simulink model "CtrPlatform_AdaptiveControl"  (Simulink 7.9)
settings: Solver=ode3  StartTime=0.0  StopTime=8  FixedStep=Ts  RelTol=1e-3
InitFcn:
  | eval('CtrPlatformCfg')
StopFcn:
  | eval('CtrPlotTrj')
values from neighbouring files (symbols this model uses):
  A = [a1 a2 a3 a4 a5 a6]/180*pi    [Config.m]    (also in CtrPlatformCfg.m)
  a2 = 0    [Config.m]    (also in CtrPlatformCfg.m)
  a3 = 0    [Config.m]    (also in CtrPlatformCfg.m)
  a4 = 0    [Config.m]    (also in CtrPlatformCfg.m)
  a5 = 90    [Config.m]    (also in CtrPlatformCfg.m)
  a6 = 0    [Config.m]    (also in CtrPlatformCfg.m)
  Cen = Cen(:)'    [Config.m]    (also in CtrPlatformCfg.m; DynEulerTest.m = Cen'; EfDynCAD.m = [cen1,cen2,cen3,cen4,cen5,cen6]')
  CurPulseFreq = 0.25*2*pi    (= 1.57079632679)    [Config.m]    (also in CtrPlatformCfg.m)
  Deg2Rad = pi/180    (= 0.0174532925199)    [Config.m]    (also in CtrPlatformCfg.m)
  DisturbSelect = 2    [Config.m]    (also in CtrPlatformCfg.m)
  DynTrjMode = 3    [Config.m]    (also in CtrPlatformCfg.m = 1)
  FbDisturbSelect = 2    [Config.m]    (also in CtrPlatformCfg.m)
  freq = tvel/radius    (= 1)    [Config.m]    (also in CtrPlatformCfg.m)
  FrictionSelect = 2    [CtrPlatformCfg.m]
  Gravity = 9.8    [Config.m]    (also in CtrPlatformCfg.m)
  Ie1 = in1(:)'    [Config.m]    (also in CtrPlatformCfg.m; DynEulerTest.m = in1(:); EfDynCAD.m = in1(:))
  Ie2 = in2(:)'    [Config.m]    (also in CtrPlatformCfg.m; DynEulerTest.m = in2(:); EfDynCAD.m = in2(:))
  Ie3 = in3(:)'    [Config.m]    (also in CtrPlatformCfg.m; DynEulerTest.m = in3(:); EfDynCAD.m = in3(:))
  Ie4 = in4(:)'    [Config.m]    (also in CtrPlatformCfg.m; DynEulerTest.m = in4(:); EfDynCAD.m = in4(:))
  Ie5 = in5(:)'    [Config.m]    (also in CtrPlatformCfg.m; DynEulerTest.m = in5(:); EfDynCAD.m = in5(:))
  Ie6 = in6(:)'    [Config.m]    (also in CtrPlatformCfg.m; DynEulerTest.m = in6(:); EfDynCAD.m = in6(:))
  in1 = [5.2954 -0.2565 -0.6366;-0.2565 4.7000 0.2830;-0.6366 0.2829 5.8635]    [Config.m]    (also in CtrPlatformCfg.m; DynEulerTest.m; EfDynCAD.m = [0.54  -0.01 0.23)
  in2 = [5.8840 0.0072 0.0135;0.0072 6.0178 -0.1907;0.0135 -0.1907 0.3374]    [Config.m]    (also in CtrPlatformCfg.m; DynEulerTest.m; EfDynCAD.m = (R_x*R_z)*in2*(R_x*R_z)')
  in3 = [1.8201 -0.2274 -0.3112;-0.2274 2.2537 -0.1441;-0.3112 -0.1441 1.9485]    [Config.m]    (also in CtrPlatformCfg.m; DynEulerTest.m; EfDynCAD.m = (R_x*R_z)*in3*(R_x*R_z)')
  in4 = [0.0607 -0.0922 0;-0.0922 1.4493 0;0 0 1.4620]    [Config.m]    (also in CtrPlatformCfg.m; DynEulerTest.m = [0.0607 -0.0922 0;-0.0922 1.4493 0;0 0,1.4620]; EfDynCAD.m = (R_y*Rz)*in4*(R_y*Rz)')
  in5 = [0.0191 0.0032 0;0.0032 0.0228 0;0 0 0.0291]    [Config.m]    (also in CtrPlatformCfg.m; DynEulerTest.m; EfDynCAD.m = (R_x*R_y)*in5*(R_x*R_y)')
  in6 = [0.0012 0 0;0 0.0007 0;0 0 0.0007]    [Config.m]    (also in CtrPlatformCfg.m; DynEulerTest.m; EfDynCAD.m = (R_y*Rz)*in6*(R_y*Rz)')
  init_Endx = gd_init(1,4)    [Config.m]    (also in CtrPlatformCfg.m)
  init_Endy = gd_init(2,4)    [Config.m]    (also in CtrPlatformCfg.m)
  init_Endz = gd_init(3,4)    [Config.m]    (also in CtrPlatformCfg.m)
  init_Rot = gd_init(1:3,1:3)    [Config.m]    (also in CtrPlatformCfg.m)
  InitialPos1 = A(1)*Rad2Line(1)    [CtrPlatformCfg.m]
  InitialPos2 = A(2)*Rad2Line(2)    [CtrPlatformCfg.m]
  InitialPos3 = A(3)*Rad2Line(3)    [CtrPlatformCfg.m]
  InitialPos4 = A(4)*Rad2Line(4)    [CtrPlatformCfg.m]
  InitialPos5 = A(5)*Rad2Line(5)    [CtrPlatformCfg.m]
  InitialPos6 = A(6)*Rad2Line(6)    [CtrPlatformCfg.m]
  JntOffset1 = A(1)    [Config.m]    (also in CtrPlatformCfg.m)
  JntOffset2 = A(2)    [Config.m]    (also in CtrPlatformCfg.m)
  JntOffset3 = A(3)    [Config.m]    (also in CtrPlatformCfg.m)
  JntOffset4 = A(4)    [Config.m]    (also in CtrPlatformCfg.m)
  JntOffset5 = A(5)    [Config.m]    (also in CtrPlatformCfg.m)
  JntOffset6 = A(6)    [Config.m]    (also in CtrPlatformCfg.m)
  L = [l1 l2 l3 l4 l5 l6 l7 l8 l9]    [Config.m]    (also in CtrPlatformCfg.m)
  LinePTs2RadpS = 2*pi/(EncRes*Ts)./Gear    [Config.m]    (also in CtrPlatformCfg.m)
  LinePTs2Rpm = 60/(EncRes*Ts)    (= 7.32421875)    [Config.m]    (also in CtrPlatformCfg.m)
  Ma = [ma1 ma2 ma3 ma4 ma5 ma6]    [Config.m]    (also in CtrPlatformCfg.m; DynEulerTest.m = [ma1; ma2; ma3; ma4; ma5; ma6]; EfDynCAD.m = [ma1 ma2 ma3 ma4 ma5 ma6]')
  ma1 = 170.31    [Config.m]    (also in CtrPlatformCfg.m; DynEulerTest.m; EfDynCAD.m = 77.75)
  ma2 = 63.74    [Config.m]    (also in CtrPlatformCfg.m; DynEulerTest.m; EfDynCAD.m = 32.31)
  ma3 = 98.98    [Config.m]    (also in CtrPlatformCfg.m; DynEulerTest.m; EfDynCAD.m = 18.61)
  ma4 = 24.46    [Config.m]    (also in CtrPlatformCfg.m; DynEulerTest.m; EfDynCAD.m = 15.65)
  ma5 = 5.24    [Config.m]    (also in CtrPlatformCfg.m; DynEulerTest.m; EfDynCAD.m = 3.32)
  ma6 = 0.6    [Config.m]    (also in CtrPlatformCfg.m; DynEulerTest.m; EfDynCAD.m)
  Pi0 = PiTest    [CtrPlatformCfg.m]
  PosPulseEnable = 1    [Config.m]    (also in CtrPlatformCfg.m)
  PosSourceSelect_Ad = 2    [CtrPlatformCfg.m]
  PosVelPulseGain = 500    [Config.m]    (also in CtrPlatformCfg.m)
  Rad2Line = Gear*EncRes/(2*pi)    [Config.m]    (also in CtrPlatformCfg.m)
  Rpm2LinePTs = EncRes*Ts/60    (= 0.136533333333)    [Config.m]    (also in CtrPlatformCfg.m)
  TrajSwitch = 1    [Config.m]    (also in CtrPlatformCfg.m)
  Trq2Cur = Trq2Cur./Cur2Trq    [Config.m]    (also in CtrPlatformCfg.m)
  Ts = 1/FrHz    (= 0.00025)    [Config.m]    (also in CtrPlatformCfg.m)
  Ts_Dyn = Ts    (= 0.00025)    [Config.m]    (also in CtrPlatformCfg.m)
  tvel = 120    [Config.m]    (also in CtrPlatformCfg.m)
  VelLpAxisNum = 1    [Config.m]    (also in CtrPlatformCfg.m)
  VelPulseEnable = 0    [Config.m]    (also in CtrPlatformCfg.m)
  VelPulseGain = 500    [Config.m]    (also in CtrPlatformCfg.m)
  Volt2Trq = Volt2Trq./Trq2Cur    [Config.m]    (also in CtrPlatformCfg.m)
undefined symbols (not defined in the file or in its folder): a1, DiscIntNeverNeededParam
libraries: simulink x56, mblibv1 x35, powerlib_extras x8, commnoisgen2 x2
(part 2 of 4)

== system CtrPlatform_AdaptiveControl/Dynamics/TrjSource ==
  Demux : Demux  Outputs=3
  DynTrjMode : Constant  Value=DynTrjMode  SampleTime=Ts_Dyn
  Multiport Switch : MultiPortSwitch  Inputs=4  zeroidx=off
  Mux : Mux  Inputs=3
  Mux1 : Mux  Inputs=3
  Mux2 : Mux  Inputs=3
  Position Loop Tunning : Subsystem
  "Robot Profile " : Subsystem
  Velocity Loop Tunning : Subsystem
  zero : Constant  Value=zeros(1,18)
  RefJntPos(Rad) : Outport
  RefJntVel(Rad/s) : Outport  Port=2
  RefJntAcc(Rad/s2) : Outport  Port=3
  wires:
  DynTrjMode/1 -> Multiport Switch/1
  "Robot Profile "/1(JntPos(Rad)) -> Mux/1
  "Robot Profile "/2(JntVel(Rad/s)) -> Mux/2
  "Robot Profile "/3(JntAcc(Rad/s2)) -> Mux/3
  Mux/1 -> Multiport Switch/2
  Velocity Loop Tunning/1(JntPos(Rad)) -> Mux1/1
  Velocity Loop Tunning/2(JntVel(Rad/s)) -> Mux1/2
  Velocity Loop Tunning/3(JntAcc(Rad/s2)) -> Mux1/3
  Mux1/1 -> Multiport Switch/3
  Position Loop Tunning/1(JntPos(Rad)) -> Mux2/1
  Position Loop Tunning/2(JntVel(Rad/s)) -> Mux2/2
  Position Loop Tunning/3(JntAcc(Rad/s2)) -> Mux2/3
  Mux2/1 -> Multiport Switch/4
  Multiport Switch/1 -> Demux/1
  Demux/3 -> RefJntAcc(Rad/s2)/1
  Demux/2 -> RefJntVel(Rad/s)/1
  Demux/1 -> RefJntPos(Rad)/1
  zero/1 -> Multiport Switch/5

== system CtrPlatform_AdaptiveControl/Fanuc/ EndSensor ==
  Avx : Scope
      settings: TimeRange=3  YMin=-150  YMax=125  SaveName=ScopeData62
  Avy : Scope
      settings: TimeRange=3  YMin=-150  YMax=125  SaveName=ScopeData63
  Avz : Scope
      settings: TimeRange=3  YMin=-150  YMax=125  SaveName=ScopeData64
  Awx : Scope
      settings: TimeRange=3  YMin=-150  YMax=125  SaveName=ScopeData65
  Awy : Scope
      settings: TimeRange=3  YMin=-150  YMax=125  SaveName=ScopeData66
  Awz : Scope
      settings: TimeRange=3  YMin=-150  YMax=125  SaveName=ScopeData67
  "Body Sensor " : mblibv1/Sensors &  Actuators/Body Sensor  UpdateFromCAD=off  PhysicalDomain=Mechanical  PortType=blob  Muxed=on  Pose=off  Angle=on  AngleUnits=deg  ArcVelocity=on  ArcVelocityUnits=deg/s  ArcAcceleration=on  ArcAccelerationUnits=deg/s^2  CoordPosition=on  CoordPositionUnits=mm  Velocity=on  VelocityUnits=mm/s  Acceleration=on  AccelerationUnits=mm/s^2  Quaternion=on  QuaternionDT=off  QuaternionDDT=off  QuaternionUnits=off  OutputVector=[1]  ActiveIO=on  Width=15  DialogClass=MechanicalSensorBlock  ReferenceFrame=Absolute (World)
  Demux5 : Demux  Outputs=15
  EndX : ToWorkspace  VariableName=EndX  SampleTime=-1  SaveFormat=Structure
  EndY : ToWorkspace  VariableName=EndY  SampleTime=-1  SaveFormat=Structure
  EndZ : ToWorkspace  VariableName=EndZ  SampleTime=-1  SaveFormat=Structure
  Vx : Scope
      settings: TimeRange=3  YMin=-150  YMax=125  SaveName=ScopeData55
  Vy : Scope
      settings: TimeRange=3  YMin=-150  YMax=125  SaveName=ScopeData57
  Vz : Scope
      settings: TimeRange=3  YMin=-150  YMax=125  SaveName=ScopeData58
  X : Scope
      settings: TimeRange=3  YMin=-150  YMax=125  SaveName=ScopeData36
  Y : Scope
      settings: TimeRange=3  YMin=-150  YMax=125  SaveName=ScopeData37
  Z : Scope
      settings: TimeRange=3  YMin=-150  YMax=125  SaveName=ScopeData38
  wx : Scope
      settings: TimeRange=3  YMin=-150  YMax=125  SaveName=ScopeData59
  wy : Scope
      settings: TimeRange=3  YMin=-150  YMax=125  SaveName=ScopeData60
  wz : Scope
      settings: TimeRange=3  YMin=-150  YMax=125  SaveName=ScopeData61
  In : PMIOPort  Port=1  Side=Left
  Out : Outport
  wires:
  "Body Sensor "/1 -> Demux5/1, Out/1
  Demux5/4 -> Vx/1
  Demux5/5 -> Vy/1
  Demux5/6 -> Vz/1
  Demux5/7 -> wx/1
  Demux5/8 -> wy/1
  Demux5/9 -> wz/1
  Demux5/10 -> Avx/1
  Demux5/11 -> Avy/1
  Demux5/12 -> Avz/1
  Demux5/13 -> Awx/1
  Demux5/14 -> Awy/1
  Demux5/15 -> Awz/1
  Demux5/1 -> EndX/1, X/1
  Demux5/2 -> EndY/1, Y/1
  Demux5/3 -> EndZ/1, Z/1
  connections:
  In/RConn1 -- "Body Sensor "/LConn1

== system CtrPlatform_AdaptiveControl/Fanuc/JointSensor1 ==
  Angle Acceleration : Scope
      settings: SaveName=ScopeData32
  Angle Velocity : Scope
      settings: SaveName=ScopeData31
  Anlge : Scope
      settings: SaveName=ScopeData30
  Computed Torque : Scope
      settings: SaveName=ScopeData33
  Demux : Demux
  Sensor1 : mblibv1/Sensors &  Actuators/Joint Sensor  UpdateFromCAD=off  PhysicalDomain=Mechanical  PortType=blob  Muxed=on  Pose=off  Angle=on  AngleUnits=deg  ArcVelocity=on  ArcVelocityUnits=deg/s  ArcAcceleration=on  ArcAccelerationUnits=deg/s^2  CoordPosition=on  CoordPositionUnits=m  Velocity=off  VelocityUnits=m/s  Acceleration=off  AccelerationUnits=m/s^2  Quaternion=on  QuaternionDT=off  QuaternionDDT=off  QuaternionUnits=off  OutputVector=[1]  ActiveIO=on  Width=4  DialogClass=MechanicalSensorBlock  Primitive=R1  Force=off  ForceUnits=N  Torque=on  TorqueUnits=N*m  ReferenceFrame=Absolute (World)  ReactionSensedSide=Follower  ReactionReferenceFrame=Absolute (World)  ReactionForce=off  ReactionForceUnits=N  ReactionMoment=off  ReactionMomentUnits=N*m
  In : PMIOPort  Port=1  Side=Left
  Out : Outport
  wires:
  Demux/4 -> Computed Torque/1
  Demux/3 -> Angle Acceleration/1
  Demux/1 -> Anlge/1
  Demux/2 -> Angle Velocity/1
  Sensor1/1 -> Out/1, Demux/1
  connections:
  In/RConn1 -- Sensor1/LConn1

== system CtrPlatform_AdaptiveControl/Fanuc/JointSensor2 ==
  Angle Acceleration : Scope
      settings: SaveName=ScopeData32
  Angle Velocity : Scope
      settings: SaveName=ScopeData31
  Anlge : Scope
      settings: SaveName=ScopeData30
  Computed Torque : Scope
      settings: SaveName=ScopeData33
  Demux : Demux
  Sensor1 : mblibv1/Sensors &  Actuators/Joint Sensor  UpdateFromCAD=off  PhysicalDomain=Mechanical  PortType=blob  Muxed=on  Pose=off  Angle=on  AngleUnits=deg  ArcVelocity=on  ArcVelocityUnits=deg/s  ArcAcceleration=on  ArcAccelerationUnits=deg/s^2  CoordPosition=on  CoordPositionUnits=m  Velocity=off  VelocityUnits=m/s  Acceleration=off  AccelerationUnits=m/s^2  Quaternion=on  QuaternionDT=off  QuaternionDDT=off  QuaternionUnits=off  OutputVector=[1]  ActiveIO=on  Width=4  DialogClass=MechanicalSensorBlock  Primitive=R1  Force=off  ForceUnits=N  Torque=on  TorqueUnits=N*m  ReferenceFrame=Absolute (World)  ReactionSensedSide=Follower  ReactionReferenceFrame=Absolute (World)  ReactionForce=off  ReactionForceUnits=N  ReactionMoment=off  ReactionMomentUnits=N*m
  In : PMIOPort  Port=1  Side=Left
  Out : Outport
  wires:
  Demux/4 -> Computed Torque/1
  Demux/3 -> Angle Acceleration/1
  Demux/1 -> Anlge/1
  Demux/2 -> Angle Velocity/1
  Sensor1/1 -> Out/1, Demux/1
  connections:
  In/RConn1 -- Sensor1/LConn1

== system CtrPlatform_AdaptiveControl/Fanuc/JointSensor3 ==
  Angle Acceleration : Scope
      settings: SaveName=ScopeData32
  Angle Velocity : Scope
      settings: SaveName=ScopeData31
  Anlge : Scope
      settings: SaveName=ScopeData30
  Computed Torque : Scope
      settings: SaveName=ScopeData33
  Demux : Demux
  Sensor1 : mblibv1/Sensors &  Actuators/Joint Sensor  UpdateFromCAD=off  PhysicalDomain=Mechanical  PortType=blob  Muxed=on  Pose=off  Angle=on  AngleUnits=deg  ArcVelocity=on  ArcVelocityUnits=deg/s  ArcAcceleration=on  ArcAccelerationUnits=deg/s^2  CoordPosition=on  CoordPositionUnits=m  Velocity=off  VelocityUnits=m/s  Acceleration=off  AccelerationUnits=m/s^2  Quaternion=on  QuaternionDT=off  QuaternionDDT=off  QuaternionUnits=off  OutputVector=[1]  ActiveIO=on  Width=4  DialogClass=MechanicalSensorBlock  Primitive=R1  Force=off  ForceUnits=N  Torque=on  TorqueUnits=N*m  ReferenceFrame=Absolute (World)  ReactionSensedSide=Follower  ReactionReferenceFrame=Absolute (World)  ReactionForce=off  ReactionForceUnits=N  ReactionMoment=off  ReactionMomentUnits=N*m
  In : PMIOPort  Port=1  Side=Left
  Out : Outport
  wires:
  Demux/4 -> Computed Torque/1
  Demux/3 -> Angle Acceleration/1
  Demux/1 -> Anlge/1
  Demux/2 -> Angle Velocity/1
  Sensor1/1 -> Out/1, Demux/1
  connections:
  In/RConn1 -- Sensor1/LConn1

== system CtrPlatform_AdaptiveControl/Fanuc/JointSensor4 ==
  Angle Acceleration : Scope
      settings: SaveName=ScopeData32
  Angle Velocity : Scope
      settings: SaveName=ScopeData31
  Anlge : Scope
      settings: SaveName=ScopeData30
  Computed Torque : Scope
      settings: SaveName=ScopeData33
  Demux : Demux
  Sensor1 : mblibv1/Sensors &  Actuators/Joint Sensor  UpdateFromCAD=off  PhysicalDomain=Mechanical  PortType=blob  Muxed=on  Pose=off  Angle=on  AngleUnits=deg  ArcVelocity=on  ArcVelocityUnits=deg/s  ArcAcceleration=on  ArcAccelerationUnits=deg/s^2  CoordPosition=on  CoordPositionUnits=m  Velocity=off  VelocityUnits=m/s  Acceleration=off  AccelerationUnits=m/s^2  Quaternion=on  QuaternionDT=off  QuaternionDDT=off  QuaternionUnits=off  OutputVector=[1]  ActiveIO=on  Width=4  DialogClass=MechanicalSensorBlock  Primitive=R1  Force=off  ForceUnits=N  Torque=on  TorqueUnits=N*m  ReferenceFrame=Absolute (World)  ReactionSensedSide=Follower  ReactionReferenceFrame=Absolute (World)  ReactionForce=off  ReactionForceUnits=N  ReactionMoment=off  ReactionMomentUnits=N*m
  In : PMIOPort  Port=1  Side=Left
  Out : Outport
  wires:
  Demux/4 -> Computed Torque/1
  Demux/3 -> Angle Acceleration/1
  Demux/1 -> Anlge/1
  Demux/2 -> Angle Velocity/1
  Sensor1/1 -> Out/1, Demux/1
  connections:
  In/RConn1 -- Sensor1/LConn1

== system CtrPlatform_AdaptiveControl/Fanuc/JointSensor5 ==
  Angle Acceleration : Scope
      settings: SaveName=ScopeData32
  Angle Velocity : Scope
      settings: SaveName=ScopeData31
  Anlge : Scope
      settings: SaveName=ScopeData30
  Computed Torque : Scope
      settings: SaveName=ScopeData33
  Demux : Demux
  Sensor1 : mblibv1/Sensors &  Actuators/Joint Sensor  UpdateFromCAD=off  PhysicalDomain=Mechanical  PortType=blob  Muxed=on  Pose=off  Angle=on  AngleUnits=deg  ArcVelocity=on  ArcVelocityUnits=deg/s  ArcAcceleration=on  ArcAccelerationUnits=deg/s^2  CoordPosition=on  CoordPositionUnits=m  Velocity=off  VelocityUnits=m/s  Acceleration=off  AccelerationUnits=m/s^2  Quaternion=on  QuaternionDT=off  QuaternionDDT=off  QuaternionUnits=off  OutputVector=[1]  ActiveIO=on  Width=4  DialogClass=MechanicalSensorBlock  Primitive=R1  Force=off  ForceUnits=N  Torque=on  TorqueUnits=N*m  ReferenceFrame=Absolute (World)  ReactionSensedSide=Follower  ReactionReferenceFrame=Absolute (World)  ReactionForce=off  ReactionForceUnits=N  ReactionMoment=off  ReactionMomentUnits=N*m
  In : PMIOPort  Port=1  Side=Left
  Out : Outport
  wires:
  Demux/4 -> Computed Torque/1
  Demux/3 -> Angle Acceleration/1
  Demux/1 -> Anlge/1
  Demux/2 -> Angle Velocity/1
  Sensor1/1 -> Out/1, Demux/1
  connections:
  In/RConn1 -- Sensor1/LConn1

== system CtrPlatform_AdaptiveControl/Fanuc/JointSensor6 ==
  Angle Acceleration : Scope
      settings: SaveName=ScopeData32
  Angle Velocity : Scope
      settings: SaveName=ScopeData31
  Anlge : Scope
      settings: SaveName=ScopeData30
  Computed Torque : Scope
      settings: SaveName=ScopeData33
  Demux : Demux
  Sensor1 : mblibv1/Sensors &  Actuators/Joint Sensor  UpdateFromCAD=off  PhysicalDomain=Mechanical  PortType=blob  Muxed=on  Pose=off  Angle=on  AngleUnits=deg  ArcVelocity=on  ArcVelocityUnits=deg/s  ArcAcceleration=on  ArcAccelerationUnits=deg/s^2  CoordPosition=on  CoordPositionUnits=m  Velocity=off  VelocityUnits=m/s  Acceleration=off  AccelerationUnits=m/s^2  Quaternion=on  QuaternionDT=off  QuaternionDDT=off  QuaternionUnits=off  OutputVector=[1]  ActiveIO=on  Width=4  DialogClass=MechanicalSensorBlock  Primitive=R1  Force=off  ForceUnits=N  Torque=on  TorqueUnits=N*m  ReferenceFrame=Absolute (World)  ReactionSensedSide=Follower  ReactionReferenceFrame=Absolute (World)  ReactionForce=off  ReactionForceUnits=N  ReactionMoment=off  ReactionMomentUnits=N*m
  In : PMIOPort  Port=1  Side=Left
  Out : Outport
  wires:
  Demux/4 -> Computed Torque/1
  Demux/3 -> Angle Acceleration/1
  Demux/1 -> Anlge/1
  Demux/2 -> Angle Velocity/1
  Sensor1/1 -> Out/1, Demux/1
  connections:
  In/RConn1 -- Sensor1/LConn1

== system CtrPlatform_AdaptiveControl/Friction Torque/Friction Torque ==
  Ff1 : Subsystem  mask{Ts=Ts, FpSelect=2}
      mask prompts: Ts "Sampling Time"
  Ff2 : Subsystem  mask{Ts=Ts, FpSelect=2}
      mask prompts: Ts "Sampling Time"
  Ff3 : Subsystem  mask{Ts=Ts, FpSelect=2}
      mask prompts: Ts "Sampling Time"
  Ff4 : Subsystem  mask{Ts=Ts, FpSelect=1}
      mask prompts: Ts "Sampling Time"
  Ff5 : Subsystem  mask{Ts=Ts, FpSelect=1}
      mask prompts: Ts "Sampling Time"
  Ff6 : Subsystem  mask{Ts=Ts, FpSelect=1}
      mask prompts: Ts "Sampling Time"
  Mux : Mux  Inputs=6
  Scope{1..6} (6 alike) : Scope
      Scope1 settings: SaveName=ScopeData70
      Scope2 settings: SaveName=ScopeData69
      Scope3 settings: SaveName=ScopeData71
      Scope4 settings: SaveName=ScopeData72
      Scope5 settings: SaveName=ScopeData73
      Scope6 settings: SaveName=ScopeData74
  Friction Torque : Outport
  wires:
  [Axis1] -> Ff1/1(dq)
  [Axis2] -> Ff2/1(dq)
  [Axis1] -> Ff3/1(dq)
  [Axis1] -> Ff4/1(dq)
  [Axis1] -> Ff5/1(dq)
  [Axis1] -> Ff6/1(dq)
  Ff1/1(Ff) -> Mux/1, Scope1/1
  Ff2/1(Ff) -> Mux/2, Scope2/1
  Ff3/1(Ff) -> Mux/3, Scope3/1
  Ff4/1(Ff) -> Mux/4, Scope4/1
  Ff5/1(Ff) -> Mux/5, Scope5/1
  Ff6/1(Ff) -> Mux/6, Scope6/1
  Mux/1 -> Friction Torque/1

== system CtrPlatform_AdaptiveControl/Signal Re-group/Re-group ==
  JntVelAcc_R1 : Inport
  Torque_R1 : Inport  Port=2
  JntVelAcc_R2 : Inport  Port=3
  Torque_R2 : Inport  Port=4
  JntVelAcc_R3 : Inport  Port=5
  Torque_R3 : Inport  Port=6
  JntVelAcc_R4 : Inport  Port=7
  Torque_R4 : Inport  Port=8
  JntVelAcc_R5 : Inport  Port=9
  Torque_R5 : Inport  Port=10
  JntVelAcc_R6 : Inport  Port=11
  Torque_R6 : Inport  Port=12
  Mux : Mux  Inputs=6
  Mux1 : Mux  Inputs=6
  JntVelAcc : Outport
  Torque : Outport  Port=2
  wires:
  JntVelAcc_R1/1 -> Mux/1
  JntVelAcc_R2/1 -> Mux/2
  JntVelAcc_R3/1 -> Mux/3
  JntVelAcc_R4/1 -> Mux/4
  JntVelAcc_R5/1 -> Mux/5
  JntVelAcc_R6/1 -> Mux/6
  Torque_R1/1 -> Mux1/1
  Torque_R2/1 -> Mux1/2
  Torque_R3/1 -> Mux1/3
  Torque_R4/1 -> Mux1/4
  Torque_R5/1 -> Mux1/5
  Torque_R6/1 -> Mux1/6
  Mux/1 -> JntVelAcc/1
  Mux1/1 -> Torque/1

== system CtrPlatform_AdaptiveControl/Signal Re-group/Re-group JntVelAcc ==
  note: Joint Angle
  note: Joint Velocity
  note: Joint Acceleration
  JntVelAcc : Inport
  Demux2 : Demux  Outputs=18
  Mux : Mux  Inputs=6
  Mux1 : Mux  Inputs=6
  Mux2 : Mux  Inputs=6
  Mux3 : Mux  Inputs=3
  ReJntVelAcc : Outport
  wires:
  JntVelAcc/1 -> Demux2/1
  Demux2/1 -> Mux/1
  Demux2/2 -> Mux1/1
  Demux2/3 -> Mux2/1
  Demux2/4 -> Mux/2
  Demux2/5 -> Mux1/2
  Demux2/6 -> Mux2/2
  Demux2/7 -> Mux/3
  Demux2/8 -> Mux1/3
  Demux2/9 -> Mux2/3
  Demux2/10 -> Mux/4
  Demux2/11 -> Mux1/4
  Demux2/12 -> Mux2/4
  Demux2/13 -> Mux/5
  Demux2/14 -> Mux1/5
  Demux2/15 -> Mux2/5
  Demux2/16 -> Mux/6
  Demux2/17 -> Mux1/6
  Demux2/18 -> Mux2/6
  Mux/1 -> Mux3/1
  Mux1/1 -> Mux3/2
  Mux2/1 -> Mux3/3
  Mux3/1 -> ReJntVelAcc/1

== system CtrPlatform_AdaptiveControl/Signal Re-group/Re-group_R1 ==
  In_R1 : Inport
  Demux2 : Demux
  Mux : Mux  Inputs=3
  JntVelAcc_R1 : Outport
  Torque_R1 : Outport  Port=2
  wires:
  In_R1/1 -> Demux2/1
  Demux2/1 -> Mux/1
  Demux2/2 -> Mux/2
  Demux2/3 -> Mux/3
  Demux2/4 -> Torque_R1/1
  Mux/1 -> JntVelAcc_R1/1

== system CtrPlatform_AdaptiveControl/Signal Re-group/Re-group_R2 ==
  In_R2 : Inport
  Demux2 : Demux
  Mux : Mux  Inputs=3
  JntVelAcc_R2 : Outport
  Torque_R2 : Outport  Port=2
  wires:
  Mux/1 -> JntVelAcc_R2/1
  Demux2/4 -> Torque_R2/1
  Demux2/3 -> Mux/3
  Demux2/2 -> Mux/2
  Demux2/1 -> Mux/1
  In_R2/1 -> Demux2/1

== system CtrPlatform_AdaptiveControl/Signal Re-group/Re-group_R3 ==
  In_R3 : Inport
  Demux2 : Demux
  Mux : Mux  Inputs=3
  JntVelAcc_R3 : Outport
  Torque_R3 : Outport  Port=2
  wires:
  In_R3/1 -> Demux2/1
  Demux2/1 -> Mux/1
  Demux2/2 -> Mux/2
  Demux2/3 -> Mux/3
  Demux2/4 -> Torque_R3/1
  Mux/1 -> JntVelAcc_R3/1

== system CtrPlatform_AdaptiveControl/Signal Re-group/Re-group_R4 ==
  In_R4 : Inport
  Demux2 : Demux
  Mux : Mux  Inputs=3
  JntVelAcc_R4 : Outport
  Torque_R4 : Outport  Port=2
  wires:
  Mux/1 -> JntVelAcc_R4/1
  Demux2/4 -> Torque_R4/1
  Demux2/3 -> Mux/3
  Demux2/2 -> Mux/2
  Demux2/1 -> Mux/1
  In_R4/1 -> Demux2/1

== system CtrPlatform_AdaptiveControl/Signal Re-group/Re-group_R5 ==
  In_R5 : Inport
  Demux2 : Demux
  Mux : Mux  Inputs=3
  JntVelAcc_R5 : Outport
  Torque_R5 : Outport  Port=2
  wires:
  In_R5/1 -> Demux2/1
  Demux2/1 -> Mux/1
  Demux2/2 -> Mux/2
  Demux2/3 -> Mux/3
  Demux2/4 -> Torque_R5/1
  Mux/1 -> JntVelAcc_R5/1

== system CtrPlatform_AdaptiveControl/Signal Re-group/Re-group_R6 ==
  In_R6 : Inport
  Demux2 : Demux
  Mux : Mux  Inputs=3
  JntVelAcc_R6 : Outport
  Torque_R6 : Outport  Port=2
  wires:
  Mux/1 -> JntVelAcc_R6/1
  Demux2/4 -> Torque_R6/1
  Demux2/3 -> Mux/3
  Demux2/2 -> Mux/2
  Demux2/1 -> Mux/1
  In_R6/1 -> Demux2/1

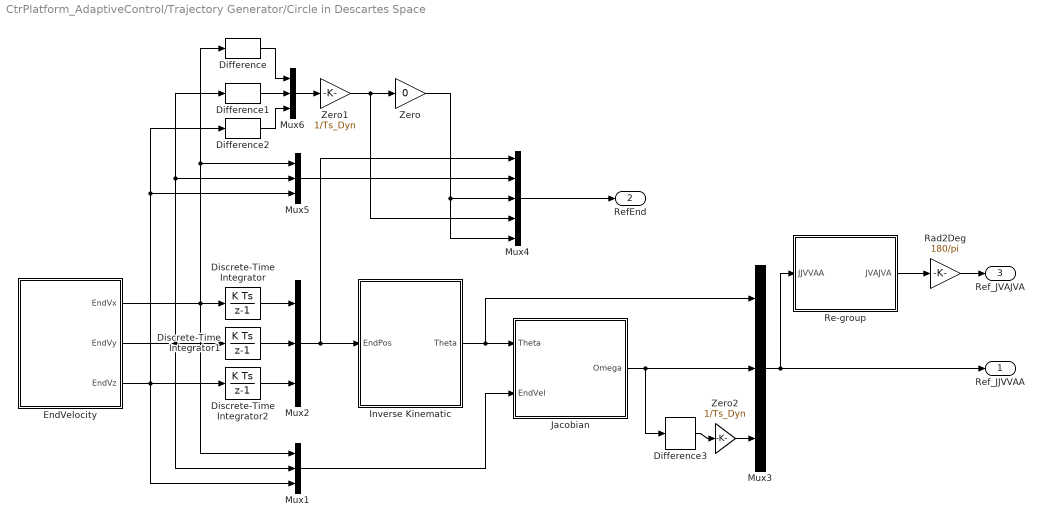
== system CtrPlatform_AdaptiveControl/Trajectory Generator/Circle in Descartes Space ==
  Difference{,1..3} (4 alike) : simulink/Discrete/Difference  ICPrevInput=0.0  InputProcessing=Inherited  OutMin=[]  OutMax=[]  OutDataType=fixdt(1, 16)  OutScaling=2^-10  DoSatur=off
  Discrete-Time Integrator : DiscreteIntegrator  InitialCondition=init_Endx  SampleTime=Ts_Dyn  ICPrevOutput=DiscIntNeverNeededParam  ICPrevScaledInput=DiscIntNeverNeededParam
  Discrete-Time Integrator1 : DiscreteIntegrator  InitialCondition=init_Endy  SampleTime=Ts_Dyn  ICPrevOutput=DiscIntNeverNeededParam  ICPrevScaledInput=DiscIntNeverNeededParam
  Discrete-Time Integrator2 : DiscreteIntegrator  InitialCondition=init_Endz  SampleTime=Ts_Dyn  ICPrevOutput=DiscIntNeverNeededParam  ICPrevScaledInput=DiscIntNeverNeededParam
  EndVelocity : Subsystem
  Inverse Kinematic : MATLAB Function  TreatAsAtomicUnit=on
  Jacobian : MATLAB Function  TreatAsAtomicUnit=on
  Mux{1..3,5..6} (5 alike) : Mux  Inputs=3
  Mux4 : Mux  Inputs=5
  Rad2Deg : Gain  Gain=180/pi
  "Re-group " : Subsystem
  Zero : Gain  Gain=0
  Zero1 : Gain  Gain=1/Ts_Dyn
  Zero2 : Gain  Gain=1/Ts_Dyn
  Ref_JJVVAA : Outport
  RefEnd : Outport  Port=2
  Ref_JVAJVA : Outport  Port=3
  wires:
  Discrete-Time Integrator/1 -> Mux2/1
  Discrete-Time Integrator1/1 -> Mux2/2
  EndVelocity/1(EndVx) -> Mux1/1, Mux5/1, Difference/1, Discrete-Time Integrator/1
  EndVelocity/2(EndVy) -> Mux1/2, Mux5/2, Difference1/1, Discrete-Time Integrator1/1
  EndVelocity/3(EndVz) -> Mux1/3, Mux5/3, Difference2/1, Discrete-Time Integrator2/1
  Discrete-Time Integrator2/1 -> Mux2/3
  Mux2/1 -> Inverse Kinematic/1(EndPos), Mux4/1
  Inverse Kinematic/1(Theta) -> Jacobian/1(Theta), Mux3/1
  Mux4/1 -> RefEnd/1
  Difference/1 -> Mux6/1
  Difference1/1 -> Mux6/2
  Difference2/1 -> Mux6/3
  Mux1/1 -> Jacobian/2(EndVel)
  Jacobian/1(Omega) -> Mux3/2, Difference3/1
  Difference3/1 -> Zero2/1
  Mux3/1 -> Ref_JJVVAA/1, "Re-group "/1(JJVVAA)
  "Re-group "/1(JVAJVA) -> Rad2Deg/1
  Mux5/1 -> Mux4/2
  Mux6/1 -> Zero1/1
  Zero/1 -> Mux4/3, Mux4/5
  Rad2Deg/1 -> Ref_JVAJVA/1
  Zero1/1 -> Mux4/4, Zero/1
  Zero2/1 -> Mux3/3

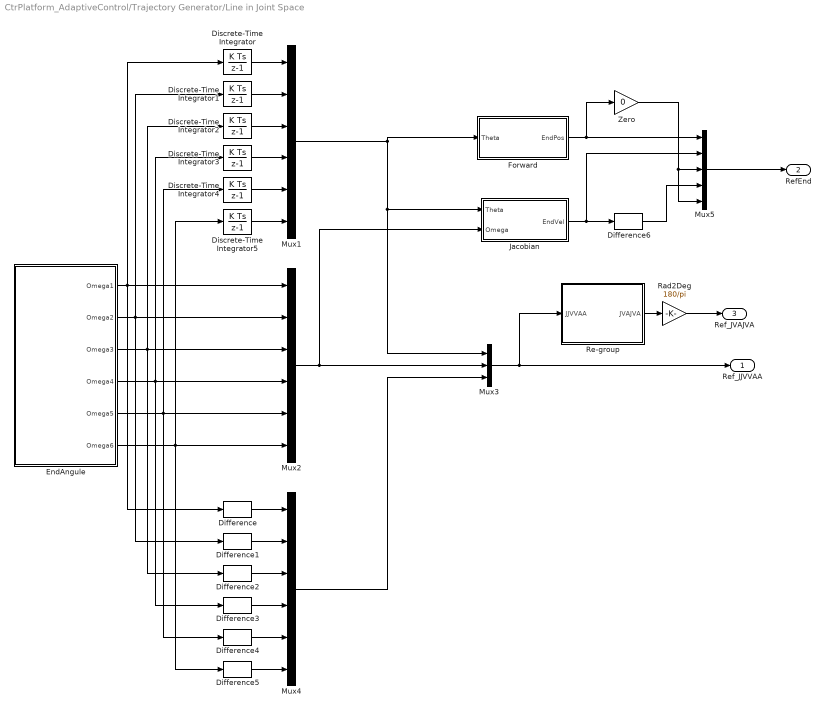
== system CtrPlatform_AdaptiveControl/Trajectory Generator/Line in Joint Space ==
  Difference{,1..6} (7 alike) : simulink/Discrete/Difference  ICPrevInput=0.0  InputProcessing=Inherited  OutMin=[]  OutMax=[]  OutDataType=fixdt(1, 16)  OutScaling=2^-10  DoSatur=off
  Discrete-Time Integrator : DiscreteIntegrator  InitialCondition=a1/180*pi  SampleTime=Ts_Dyn  ICPrevOutput=DiscIntNeverNeededParam  ICPrevScaledInput=DiscIntNeverNeededParam
  Discrete-Time Integrator1 : DiscreteIntegrator  InitialCondition=a2/180*pi  SampleTime=Ts_Dyn  ICPrevOutput=DiscIntNeverNeededParam  ICPrevScaledInput=DiscIntNeverNeededParam
  Discrete-Time Integrator2 : DiscreteIntegrator  InitialCondition=a3/180*pi  SampleTime=Ts_Dyn  ICPrevOutput=DiscIntNeverNeededParam  ICPrevScaledInput=DiscIntNeverNeededParam
  Discrete-Time Integrator3 : DiscreteIntegrator  InitialCondition=a4/180*pi  SampleTime=Ts_Dyn  ICPrevOutput=DiscIntNeverNeededParam  ICPrevScaledInput=DiscIntNeverNeededParam
  Discrete-Time Integrator4 : DiscreteIntegrator  InitialCondition=a5/180*pi  SampleTime=Ts_Dyn  ICPrevOutput=DiscIntNeverNeededParam  ICPrevScaledInput=DiscIntNeverNeededParam
  Discrete-Time Integrator5 : DiscreteIntegrator  InitialCondition=a6/180*pi  SampleTime=Ts_Dyn  ICPrevOutput=DiscIntNeverNeededParam  ICPrevScaledInput=DiscIntNeverNeededParam
  EndAngule : Subsystem
  Forward : MATLAB Function  TreatAsAtomicUnit=on
  Jacobian : MATLAB Function  TreatAsAtomicUnit=on
  Mux1 : Mux  Inputs=6
  Mux2 : Mux  Inputs=6
  Mux3 : Mux  Inputs=3
  Mux4 : Mux  Inputs=6
  Mux5 : Mux  Inputs=5
  Rad2Deg : Gain  Gain=180/pi
  "Re-group " : Subsystem
  Zero : Gain  Gain=0
  Ref_JJVVAA : Outport
  RefEnd : Outport  Port=2
  Ref_JVAJVA : Outport  Port=3
  wires:
  Forward/1(EndPos) -> Mux5/1, Zero/1
  Mux5/1 -> RefEnd/1
  Mux4/1 -> Mux3/3
  Mux1/1 -> Jacobian/1(Theta), Mux3/1, Forward/1(Theta)
  Mux2/1 -> Jacobian/2(Omega), Mux3/2
  Difference5/1 -> Mux4/6
  Difference4/1 -> Mux4/5
  Difference3/1 -> Mux4/4
  Difference2/1 -> Mux4/3
  Difference1/1 -> Mux4/2
  Difference/1 -> Mux4/1
  Discrete-Time Integrator5/1 -> Mux1/6
  Discrete-Time Integrator4/1 -> Mux1/5
  Discrete-Time Integrator3/1 -> Mux1/4
  Discrete-Time Integrator2/1 -> Mux1/3
  Discrete-Time Integrator1/1 -> Mux1/2
  Discrete-Time Integrator/1 -> Mux1/1
  EndAngule/6(Omega6) -> Mux2/6, Discrete-Time Integrator5/1, Difference5/1
  EndAngule/5(Omega5) -> Mux2/5, Discrete-Time Integrator4/1, Difference4/1
  EndAngule/4(Omega4) -> Mux2/4, Discrete-Time Integrator3/1, Difference3/1
  EndAngule/3(Omega3) -> Mux2/3, Discrete-Time Integrator2/1, Difference2/1
  EndAngule/2(Omega2) -> Mux2/2, Discrete-Time Integrator1/1, Difference1/1
  EndAngule/1(Omega1) -> Mux2/1, Discrete-Time Integrator/1, Difference/1
  Mux3/1 -> Ref_JJVVAA/1, "Re-group "/1(JJVVAA)
  "Re-group "/1(JVAJVA) -> Rad2Deg/1
  Jacobian/1(EndVel) -> Mux5/2, Difference6/1
  Difference6/1 -> Mux5/4
  Zero/1 -> Mux5/3, Mux5/5
  Rad2Deg/1 -> Ref_JVAJVA/1

== system CtrPlatform_AdaptiveControl/Trajectory Generator/Still ==
  Difference{,1..3} (4 alike) : simulink/Discrete/Difference  ICPrevInput=0.0  InputProcessing=Inherited  OutMin=[]  OutMax=[]  OutDataType=fixdt(1, 16)  OutScaling=2^-10  DoSatur=off
  Discrete-Time Integrator : DiscreteIntegrator  InitialCondition=init_Endx  SampleTime=Ts_Dyn  ICPrevOutput=DiscIntNeverNeededParam  ICPrevScaledInput=DiscIntNeverNeededParam
  Discrete-Time Integrator1 : DiscreteIntegrator  InitialCondition=init_Endy  SampleTime=Ts_Dyn  ICPrevOutput=DiscIntNeverNeededParam  ICPrevScaledInput=DiscIntNeverNeededParam
  Discrete-Time Integrator2 : DiscreteIntegrator  InitialCondition=init_Endz  SampleTime=Ts_Dyn  ICPrevOutput=DiscIntNeverNeededParam  ICPrevScaledInput=DiscIntNeverNeededParam
  EndVelocity : Subsystem
  Inverse Kinematic : MATLAB Function  TreatAsAtomicUnit=on
  Jacobian : MATLAB Function  TreatAsAtomicUnit=on
  Mux{1..3,5..6} (5 alike) : Mux  Inputs=3
  Mux4 : Mux  Inputs=5
  Rad2Deg : Gain  Gain=180/pi
  "Re-group " : Subsystem
  Zero : Gain  Gain=0
  Ref_JJVVAA : Outport
  RefEnd : Outport  Port=2
  Ref_JVAJVA : Outport  Port=3
  wires:
  Zero/1 -> Mux4/5, Mux4/3
  Mux6/1 -> Zero/1, Mux4/4
  Mux5/1 -> Mux4/2
  "Re-group "/1(JVAJVA) -> Rad2Deg/1
  Mux3/1 -> "Re-group "/1(JJVVAA), Ref_JJVVAA/1
  Difference3/1 -> Mux3/3
  Jacobian/1(Omega) -> Mux3/2, Difference3/1
  Mux1/1 -> Jacobian/2(EndVel)
  Difference2/1 -> Mux6/3
  Difference1/1 -> Mux6/2
  Difference/1 -> Mux6/1
  Mux4/1 -> RefEnd/1
  Inverse Kinematic/1(Theta) -> Mux3/1, Jacobian/1(Theta)
  Mux2/1 -> Mux4/1, Inverse Kinematic/1(EndPos)
  Discrete-Time Integrator2/1 -> Mux2/3
  EndVelocity/3(EndVz) -> Mux5/3, Difference2/1, Mux1/3, Discrete-Time Integrator2/1
  EndVelocity/2(EndVy) -> Mux5/2, Difference1/1, Mux1/2, Discrete-Time Integrator1/1
  EndVelocity/1(EndVx) -> Mux5/1, Difference/1, Mux1/1, Discrete-Time Integrator/1
  Discrete-Time Integrator1/1 -> Mux2/2
  Discrete-Time Integrator/1 -> Mux2/1
  Rad2Deg/1 -> Ref_JVAJVA/1

== system CtrPlatform_AdaptiveControl/Controller/Diff2Vel1/Filters ==
  In : Inport
  Demux : Demux  Outputs=6
  Discrete  2nd-Order Filter{,1..5} (6 alike) : powerlib_extras/Discrete  Control Blocks/Discrete  2nd-Order Filter  FilterType=Lowpass  Fo=200  Zeta=0.707  Ts=Ts  Initialize=off  Vac_Init=[0.8 -25 60]  Vdc_Init=-0.4  PlotResponse=off  param1=[1 500 1]
  Mux : Mux  Inputs=6
  Out : Outport
  wires:
  Demux/1 -> Discrete  2nd-Order Filter/1
  Demux/2 -> Discrete  2nd-Order Filter1/1
  Demux/3 -> Discrete  2nd-Order Filter2/1
  Demux/4 -> Discrete  2nd-Order Filter3/1
  Demux/5 -> Discrete  2nd-Order Filter4/1
  Demux/6 -> Discrete  2nd-Order Filter5/1
  Discrete  2nd-Order Filter/1 -> Mux/1
  Discrete  2nd-Order Filter1/1 -> Mux/2
  Discrete  2nd-Order Filter2/1 -> Mux/3
  Discrete  2nd-Order Filter3/1 -> Mux/4
  Discrete  2nd-Order Filter4/1 -> Mux/5
  Discrete  2nd-Order Filter5/1 -> Mux/6
  In/1 -> Demux/1
  Mux/1 -> Out/1

== system CtrPlatform_AdaptiveControl/Controller/Pi_Observe/s1 ==
  In1 : Inport
  Demux3 : Demux  Outputs=6
  Scope{8..13} (6 alike) : Scope
      Scope10 settings: SaveName=ScopeData78
      Scope11 settings: SaveName=ScopeData81
      Scope12 settings: SaveName=ScopeData82
      Scope13 settings: SaveName=ScopeData83
      Scope8 settings: SaveName=ScopeData84
      Scope9 settings: SaveName=ScopeData85
  wires:
  Demux3/1 -> Scope9/1
  Demux3/2 -> Scope10/1
  Demux3/3 -> Scope11/1
  Demux3/5 -> Scope12/1
  Demux3/6 -> Scope13/1
  Demux3/4 -> Scope8/1
  In1/1 -> Demux3/1

== system CtrPlatform_AdaptiveControl/Controller/Pi_Observe/s10 ==
  In1 : Inport
  Demux3 : Demux  Outputs=6
  Scope{8..13} (6 alike) : Scope
      Scope10 settings: SaveName=ScopeData78
      Scope11 settings: SaveName=ScopeData81
      Scope12 settings: SaveName=ScopeData82
      Scope13 settings: SaveName=ScopeData83
      Scope8 settings: SaveName=ScopeData84
      Scope9 settings: SaveName=ScopeData85
  wires:
  Demux3/1 -> Scope9/1
  Demux3/2 -> Scope10/1
  Demux3/3 -> Scope11/1
  Demux3/5 -> Scope12/1
  Demux3/6 -> Scope13/1
  Demux3/4 -> Scope8/1
  In1/1 -> Demux3/1

== system CtrPlatform_AdaptiveControl/Controller/Pi_Observe/s2 ==
  In1 : Inport
  Demux3 : Demux  Outputs=6
  Scope{8..13} (6 alike) : Scope
      Scope10 settings: SaveName=ScopeData78
      Scope11 settings: SaveName=ScopeData81
      Scope12 settings: SaveName=ScopeData82
      Scope13 settings: SaveName=ScopeData83
      Scope8 settings: SaveName=ScopeData84
      Scope9 settings: SaveName=ScopeData85
  wires:
  Demux3/1 -> Scope9/1
  Demux3/2 -> Scope10/1
  Demux3/3 -> Scope11/1
  Demux3/5 -> Scope12/1
  Demux3/6 -> Scope13/1
  Demux3/4 -> Scope8/1
  In1/1 -> Demux3/1

== system CtrPlatform_AdaptiveControl/Controller/Pi_Observe/s3 ==
  In1 : Inport
  Demux3 : Demux  Outputs=6
  Scope{8..13} (6 alike) : Scope
      Scope10 settings: SaveName=ScopeData78
      Scope11 settings: SaveName=ScopeData81
      Scope12 settings: SaveName=ScopeData82
      Scope13 settings: SaveName=ScopeData83
      Scope8 settings: SaveName=ScopeData84
      Scope9 settings: SaveName=ScopeData85
  wires:
  Demux3/1 -> Scope9/1
  Demux3/2 -> Scope10/1
  Demux3/3 -> Scope11/1
  Demux3/5 -> Scope12/1
  Demux3/6 -> Scope13/1
  Demux3/4 -> Scope8/1
  In1/1 -> Demux3/1

== system CtrPlatform_AdaptiveControl/Controller/Pi_Observe/s4 ==
  In1 : Inport
  Demux3 : Demux  Outputs=6
  Scope{8..13} (6 alike) : Scope
      Scope10 settings: SaveName=ScopeData78
      Scope11 settings: SaveName=ScopeData81
      Scope12 settings: SaveName=ScopeData82
      Scope13 settings: SaveName=ScopeData83
      Scope8 settings: SaveName=ScopeData84
      Scope9 settings: SaveName=ScopeData85
  wires:
  Demux3/1 -> Scope9/1
  Demux3/2 -> Scope10/1
  Demux3/3 -> Scope11/1
  Demux3/5 -> Scope12/1
  Demux3/6 -> Scope13/1
  Demux3/4 -> Scope8/1
  In1/1 -> Demux3/1

== system CtrPlatform_AdaptiveControl/Controller/Pi_Observe/s5 ==
  In1 : Inport
  Demux3 : Demux  Outputs=6
  Scope{8..13} (6 alike) : Scope
      Scope10 settings: SaveName=ScopeData78
      Scope11 settings: SaveName=ScopeData81
      Scope12 settings: SaveName=ScopeData82
      Scope13 settings: SaveName=ScopeData83
      Scope8 settings: SaveName=ScopeData84
      Scope9 settings: SaveName=ScopeData85
  wires:
  Demux3/1 -> Scope9/1
  Demux3/2 -> Scope10/1
  Demux3/3 -> Scope11/1
  Demux3/5 -> Scope12/1
  Demux3/6 -> Scope13/1
  Demux3/4 -> Scope8/1
  In1/1 -> Demux3/1

== system CtrPlatform_AdaptiveControl/Controller/Pi_Observe/s6 ==
  In1 : Inport
  Demux3 : Demux  Outputs=6
  Scope{8..13} (6 alike) : Scope
      Scope10 settings: SaveName=ScopeData78
      Scope11 settings: SaveName=ScopeData81
      Scope12 settings: SaveName=ScopeData82
      Scope13 settings: SaveName=ScopeData83
      Scope8 settings: SaveName=ScopeData84
      Scope9 settings: SaveName=ScopeData85
  wires:
  Demux3/1 -> Scope9/1
  Demux3/2 -> Scope10/1
  Demux3/3 -> Scope11/1
  Demux3/5 -> Scope12/1
  Demux3/6 -> Scope13/1
  Demux3/4 -> Scope8/1
  In1/1 -> Demux3/1

== system CtrPlatform_AdaptiveControl/Controller/Pi_Observe/s7 ==
  In1 : Inport
  Demux3 : Demux  Outputs=6
  Scope{8..13} (6 alike) : Scope
      Scope10 settings: SaveName=ScopeData78
      Scope11 settings: SaveName=ScopeData81
      Scope12 settings: SaveName=ScopeData82
      Scope13 settings: SaveName=ScopeData83
      Scope8 settings: SaveName=ScopeData84
      Scope9 settings: SaveName=ScopeData85
  wires:
  Demux3/1 -> Scope9/1
  Demux3/2 -> Scope10/1
  Demux3/3 -> Scope11/1
  Demux3/5 -> Scope12/1
  Demux3/6 -> Scope13/1
  Demux3/4 -> Scope8/1
  In1/1 -> Demux3/1

== system CtrPlatform_AdaptiveControl/Controller/Pi_Observe/s8 ==
  In1 : Inport
  Demux3 : Demux  Outputs=6
  Scope{8..13} (6 alike) : Scope
      Scope10 settings: SaveName=ScopeData78
      Scope11 settings: SaveName=ScopeData81
      Scope12 settings: SaveName=ScopeData82
      Scope13 settings: SaveName=ScopeData83
      Scope8 settings: SaveName=ScopeData84
      Scope9 settings: SaveName=ScopeData85
  wires:
  Demux3/1 -> Scope9/1
  Demux3/2 -> Scope10/1
  Demux3/3 -> Scope11/1
  Demux3/5 -> Scope12/1
  Demux3/6 -> Scope13/1
  Demux3/4 -> Scope8/1
  In1/1 -> Demux3/1

== system CtrPlatform_AdaptiveControl/Controller/Pi_Observe/s9 ==
  In1 : Inport
  Demux3 : Demux  Outputs=6
  Scope{8..13} (6 alike) : Scope
      Scope10 settings: SaveName=ScopeData78
      Scope11 settings: SaveName=ScopeData81
      Scope12 settings: SaveName=ScopeData82
      Scope13 settings: SaveName=ScopeData83
      Scope8 settings: SaveName=ScopeData84
      Scope9 settings: SaveName=ScopeData85
  wires:
  Demux3/1 -> Scope9/1
  Demux3/2 -> Scope10/1
  Demux3/3 -> Scope11/1
  Demux3/5 -> Scope12/1
  Demux3/6 -> Scope13/1
  Demux3/4 -> Scope8/1
  In1/1 -> Demux3/1

== system CtrPlatform_AdaptiveControl/Controller/Source Model/PosVel Pulse Cmd ==
  Enable : Inport
  Add1 : Sum
  CmdVel(rpm) : Scope
      settings: SaveName=ScopeData2
  Data Type  Conversion : DataTypeConversion  OutDataTypeStr=uint8  SaturateOnIntegerOverflow=on  RndMeth=Zero
  Discrete  2nd-Order Filter : powerlib_extras/Discrete  Control Blocks/Discrete  2nd-Order Filter  FilterType=Lowpass  Fo=10  Zeta=0.9  Ts=Ts_Dyn  Initialize=off  Vac_Init=[0.8 -25 60]  Vdc_Init=-0.4  PlotResponse=off  param1=[1 500 1]
  LinePTs2Rpm : Gain  Gain=LinePTs2Rpm
  Logical Operator : Logic  Operator=NOT  AllPortsSameDT=off  OutDataTypeStr=boolean
  Logical Operator1 : Logic  Operator=OR  AllPortsSameDT=off  OutDataTypeStr=boolean
  Multiport Switch : MultiPortSwitch  Inputs=2  zeroidx=off
  One : Constant  OutDataTypeStr=boolean  SampleTime=Ts_Dyn
  Pulse Generator : Subsystem
  Triggered Subsystem : Subsystem  TreatAsAtomicUnit=on
  Zero Refrence : Subsystem
  Cmd(LpTs) : Outport
  wires:
  LinePTs2Rpm/1 -> CmdVel(rpm)/1
  Logical Operator/1 -> Logical Operator1/1
  Zero Refrence/1(Pulse) -> Multiport Switch/3
  Pulse Generator/1(Pulse(LinePTs)) -> Multiport Switch/2
  One/1 -> Add1/2
  Add1/1 -> Multiport Switch/1
  Data Type  Conversion/1 -> Add1/1
  Multiport Switch/1 -> Discrete  2nd-Order Filter/1
  Enable/1 -> Logical Operator/1, Pulse Generator/Enable
  Logical Operator1/1 -> Data Type  Conversion/1, Zero Refrence/Enable
  Triggered Subsystem/1(Out1) -> Logical Operator1/2
  Discrete  2nd-Order Filter/1 -> LinePTs2Rpm/1, Cmd(LpTs)/1
  Pulse Generator/2(TimePulse) -> Triggered Subsystem/Trigger

== system CtrPlatform_AdaptiveControl/Controller/Source Model/Vel Pulse Cmd ==
  Enable : Inport
  Add1 : Sum
  CmdVel(rpm) : Scope
      settings: SaveName=ScopeData2
  Data Type  Conversion : DataTypeConversion  OutDataTypeStr=uint8  SaturateOnIntegerOverflow=on  RndMeth=Zero
  Discrete  2nd-Order Filter : powerlib_extras/Discrete  Control Blocks/Discrete  2nd-Order Filter  FilterType=Lowpass  Fo=10  Zeta=0.9  Ts=Ts_Dyn  Initialize=off  Vac_Init=[0.8 -25 60]  Vdc_Init=-0.4  PlotResponse=off  param1=[1 500 1]
  LinePTs2Rpm : Gain  Gain=LinePTs2Rpm
  Logical Operator : Logic  Operator=NOT  AllPortsSameDT=off  OutDataTypeStr=boolean
  Logical Operator1 : Logic  Operator=OR  AllPortsSameDT=off  OutDataTypeStr=boolean
  Multiport Switch : MultiPortSwitch  Inputs=2  zeroidx=off
  One : Constant  OutDataTypeStr=boolean  SampleTime=Ts_Dyn
  Pulse Generator : Subsystem
  Triggered Subsystem : Subsystem  TreatAsAtomicUnit=on
  Zero Refrence : Subsystem
  Cmd(LpTs) : Outport
  wires:
  Pulse Generator/2(TimePulse) -> Triggered Subsystem/Trigger
  Discrete  2nd-Order Filter/1 -> Cmd(LpTs)/1, LinePTs2Rpm/1
  Triggered Subsystem/1(Out1) -> Logical Operator1/2
  Logical Operator1/1 -> Zero Refrence/Enable, Data Type  Conversion/1
  Enable/1 -> Pulse Generator/Enable, Logical Operator/1
  Multiport Switch/1 -> Discrete  2nd-Order Filter/1
  Data Type  Conversion/1 -> Add1/1
  Add1/1 -> Multiport Switch/1
  One/1 -> Add1/2
  Pulse Generator/1(Pulse(LinePTs)) -> Multiport Switch/2
  Zero Refrence/1(Pulse) -> Multiport Switch/3
  Logical Operator/1 -> Logical Operator1/1
  LinePTs2Rpm/1 -> CmdVel(rpm)/1

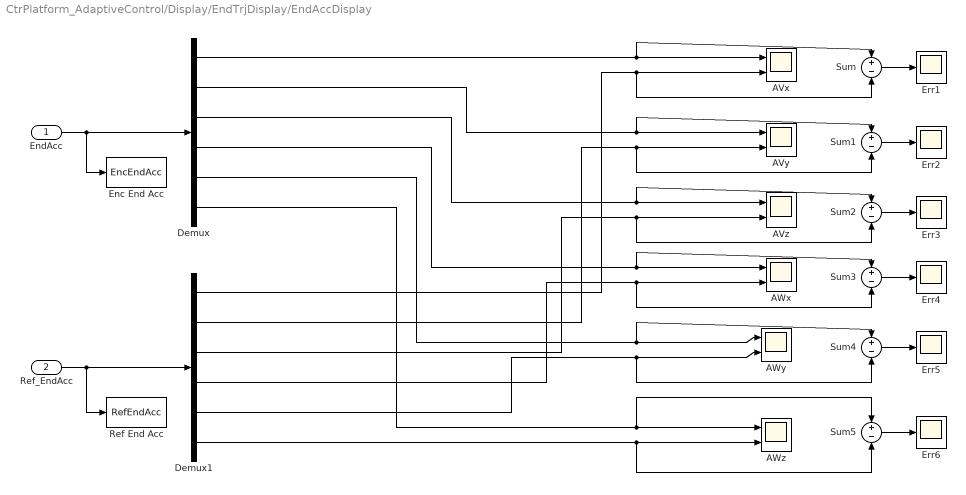
== system CtrPlatform_AdaptiveControl/Display/EndTrjDisplay/EndAccDisplay ==
  EndAcc : Inport
  Ref_EndAcc : Inport  Port=2
  AVx : Scope  NumInputPorts=2
      settings: TimeRange=10  YMin=-2.999999999999999e-017~-1  YMax=4e-017~1
  "AVy " : Scope  NumInputPorts=2
      settings: YMin=-5~-5  YMax=5~5
  AVz : Scope  NumInputPorts=2
      settings: YMin=-5~-5  YMax=5~5  SaveName=ScopeData2
  AWx : Scope  NumInputPorts=2
      settings: YMin=-5~-5  YMax=5~5  SaveName=ScopeData3
  AWy : Scope  NumInputPorts=2
      settings: TimeRange=10  YMin=-4.18~4.060000000000001  YMax=-4.04~4.2  SaveName=ScopeData4
  AWz : Scope  NumInputPorts=2
      settings: TimeRange=10  YMin=-1.6e-006~-0.003  YMax=4e-007~0.004  SaveName=ScopeData5
  Demux : Demux  Outputs=6
  Demux1 : Demux  Outputs=6
  Enc End Acc : ToWorkspace  VariableName=EncEndAcc  SampleTime=-1  SaveFormat=Structure
  Err{1..6} (6 alike) : Scope
      Err1 settings: SaveName=ScopeData6
      Err2 settings: SaveName=ScopeData7
      Err3 settings: SaveName=ScopeData8
      Err4 settings: SaveName=ScopeData9
      Err5 settings: TimeRange=3  YMin=-2.5  YMax=1  SaveName=ScopeData10
      Err6 settings: SaveName=ScopeData11
  Ref End Acc : ToWorkspace  VariableName=RefEndAcc  SampleTime=-1  SaveFormat=Structure
  Sum{,1..5} (6 alike) : Sum  Inputs=+|-
  wires:
  Sum/1 -> Err1/1
  Sum1/1 -> Err2/1
  Sum2/1 -> Err3/1
  Sum3/1 -> Err4/1
  Sum4/1 -> Err5/1
  Sum5/1 -> Err6/1
  EndAcc/1 -> Demux/1, Enc End Acc/1
  Ref_EndAcc/1 -> Demux1/1, Ref End Acc/1
  Demux/1 -> Sum/1, AVx/1
  Demux1/1 -> Sum/2, AVx/2
  Demux/2 -> "AVy "/1, Sum1/1
  Demux/3 -> AVz/1, Sum2/1
  Demux/4 -> Sum3/1, AWx/1
  Demux/5 -> AWy/1, Sum4/1
  Demux/6 -> AWz/1, Sum5/1
  Demux1/2 -> "AVy "/2, Sum1/2
  Demux1/3 -> AVz/2, Sum2/2
  Demux1/4 -> Sum3/2, AWx/2
  Demux1/5 -> AWy/2, Sum4/2
  Demux1/6 -> AWz/2, Sum5/2

== system CtrPlatform_AdaptiveControl/Display/EndTrjDisplay/EndPosDisplay ==
  EndPos : Inport
  Ref_EndPos : Inport  Port=2
  Demux : Demux  Outputs=3
  Demux1 : Demux  Outputs=3
  "Encoder " : ToWorkspace  VariableName=EncEndPos  SampleTime=-1  SaveFormat=Structure
  Err1 : Scope
      settings: SaveName=ScopeData6
  Err2 : Scope
      settings: SaveName=ScopeData7
  Err3 : Scope
      settings: SaveName=ScopeData8
  Mux : Mux  Inputs=2
  Mux1 : Mux  Inputs=2
  Mux2 : Mux  Inputs=2
  "Ref " : ToWorkspace  VariableName=RefEndPos  SampleTime=-1  SaveFormat=Structure
  Sum : Sum  Inputs=+|-
  Sum1 : Sum  Inputs=+|-
  Sum2 : Sum  Inputs=+|-
  X : Scope
      settings: TimeRange=5  YMin=1166  YMax=1166  SaveName=EndPosX
  "Y " : Scope
      settings: YMin=5  YMax=55  SaveName=EndPosY
  Z : Scope
      settings: SaveName=EndPosZ
  wires:
  Ref_EndPos/1 -> "Ref "/1, Demux1/1
  EndPos/1 -> "Encoder "/1, Demux/1
  Sum2/1 -> Err3/1
  Sum1/1 -> Err2/1
  Sum/1 -> Err1/1
  Demux/1 -> Sum/1, Mux/1
  Demux1/1 -> Sum/2, Mux/2
  Demux/2 -> Sum1/1, Mux1/1
  Demux1/2 -> Sum1/2, Mux1/2
  Demux/3 -> Sum2/1, Mux2/1
  Demux1/3 -> Sum2/2, Mux2/2
  Mux/1 -> X/1
  Mux1/1 -> "Y "/1
  Mux2/1 -> Z/1

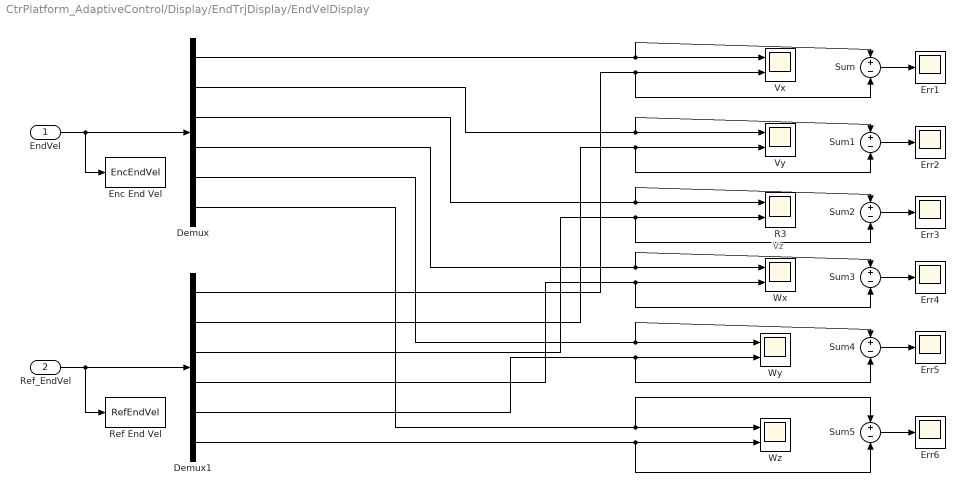
== system CtrPlatform_AdaptiveControl/Display/EndTrjDisplay/EndVelDisplay ==
  note: Vz
  EndVel : Inport
  Ref_EndVel : Inport  Port=2
  Demux : Demux  Outputs=6
  Demux1 : Demux  Outputs=6
  Enc End Vel : ToWorkspace  VariableName=EncEndVel  SampleTime=-1  SaveFormat=Structure
  Err{1..6} (6 alike) : Scope
      Err1 settings: SaveName=ScopeData6
      Err2 settings: SaveName=ScopeData7
      Err3 settings: SaveName=ScopeData8
      Err4 settings: SaveName=ScopeData9
      Err5 settings: TimeRange=3  YMin=-2.5  YMax=1  SaveName=ScopeData10
      Err6 settings: SaveName=ScopeData11
  R3 : Scope  NumInputPorts=2
      settings: YMin=-5~-5  YMax=5~5  SaveName=ScopeData2
  Ref End Vel : ToWorkspace  VariableName=RefEndVel  SampleTime=-1  SaveFormat=Structure
  Sum{,1..5} (6 alike) : Sum  Inputs=+|-
  Vx : Scope  NumInputPorts=2
      settings: TimeRange=1  YMin=-400~-1  YMax=1200~1
  "Vy " : Scope  NumInputPorts=2
      settings: YMin=-5~-5  YMax=5~5
  Wx : Scope  NumInputPorts=2
      settings: YMin=-5~-5  YMax=5~5  SaveName=ScopeData3
  Wy : Scope  NumInputPorts=2
      settings: TimeRange=10  YMin=-4.18~4.060000000000001  YMax=-4.04~4.2  SaveName=ScopeData4
  Wz : Scope  NumInputPorts=2
      settings: TimeRange=10  YMin=-1.6e-006~-0.003  YMax=4e-007~0.004  SaveName=ScopeData5
  wires:
  Demux1/6 -> Sum5/2, Wz/2
  Demux1/5 -> Sum4/2, Wy/2
  Demux1/4 -> Wx/2, Sum3/2
  Demux1/3 -> Sum2/2, R3/2
  Demux1/2 -> Sum1/2, "Vy "/2
  Demux/6 -> Sum5/1, Wz/1
  Demux/5 -> Sum4/1, Wy/1
  Demux/4 -> Wx/1, Sum3/1
  Demux/3 -> Sum2/1, R3/1
  Demux/2 -> Sum1/1, "Vy "/1
  Demux1/1 -> Vx/2, Sum/2
  Demux/1 -> Vx/1, Sum/1
  Ref_EndVel/1 -> Ref End Vel/1, Demux1/1
  EndVel/1 -> Enc End Vel/1, Demux/1
  Sum5/1 -> Err6/1
  Sum4/1 -> Err5/1
  Sum3/1 -> Err4/1
  Sum2/1 -> Err3/1
  Sum1/1 -> Err2/1
  Sum/1 -> Err1/1

== system CtrPlatform_AdaptiveControl/Display/JntVelAccDisplay/Joint1 ==
  JVA1 : Inport
  Ref_JVA1 : Inport  Port=2
  Acceleration : Scope
      settings: YMin=-5.76  YMax=-5.69  SaveName=ScopeData54
  Angle : Scope
      settings: TimeRange=8  YMin=8.025  YMax=8.575  SaveName=ScopeData52
  Demux : Demux  Outputs=3
  Demux1 : Demux  Outputs=3
  "Encoder " : ToWorkspace  VariableName=EncJVAJ1  SampleTime=-1  SaveFormat=Structure
  Err1 : Scope
      settings: SaveName=ScopeData6
  Err2 : Scope
      settings: SaveName=ScopeData7
  Err3 : Scope
      settings: SaveName=ScopeData8
  Mux : Mux  Inputs=2
  Mux1 : Mux  Inputs=2
  Mux2 : Mux  Inputs=2
  "Ref " : ToWorkspace  VariableName=RefJVAJ1  SampleTime=-1  SaveFormat=Structure
  Sum : Sum  Inputs=+|-
  Sum1 : Sum  Inputs=+|-
  Sum2 : Sum  Inputs=+|-
  "Velocity " : Scope
      settings: YMin=0.35  YMax=1.05  SaveName=ScopeData53
  wires:
  Ref_JVA1/1 -> "Ref "/1, Demux1/1
  JVA1/1 -> "Encoder "/1, Demux/1
  Sum2/1 -> Err3/1
  Sum1/1 -> Err2/1
  Sum/1 -> Err1/1
  Demux/1 -> Sum/1, Mux/1
  Demux1/1 -> Sum/2, Mux/2
  Demux/2 -> Sum1/1, Mux1/1
  Demux1/2 -> Sum1/2, Mux1/2
  Demux/3 -> Sum2/1, Mux2/1
  Demux1/3 -> Sum2/2, Mux2/2
  Mux/1 -> Angle/1
  Mux1/1 -> "Velocity "/1
  Mux2/1 -> Acceleration/1

== system CtrPlatform_AdaptiveControl/Display/JntVelAccDisplay/Joint2 ==
  JVA2 : Inport
  Ref_JVA2 : Inport  Port=2
  Acceleration : Scope  NumInputPorts=2
      settings: YMin=0.0255~-0.599  YMax=0.03125~-0.581  SaveName=ScopeData2
  Angle : Scope  NumInputPorts=2
      settings: YMin=-9.5~-0.3  YMax=-6.5~-0.225
  Demux : Demux  Outputs=3
  Demux1 : Demux  Outputs=3
  "Encoder " : ToWorkspace  VariableName=EncJVAJ2  SampleTime=-1  SaveFormat=Structure
  Err1 : Scope
      settings: SaveName=ScopeData6
  Err2 : Scope
      settings: SaveName=ScopeData7
  Err3 : Scope
      settings: SaveName=ScopeData8
  "Ref " : ToWorkspace  VariableName=RefJVAJ2  SampleTime=-1  SaveFormat=Structure
  Sum : Sum  Inputs=+|-
  Sum1 : Sum  Inputs=+|-
  Sum2 : Sum  Inputs=+|-
  "Velocity " : Scope  NumInputPorts=2
      settings: YMin=0.00875~0.17  YMax=0.0097~0.205
  wires:
  Demux1/3 -> Sum2/2, Acceleration/2
  Demux/3 -> Sum2/1, Acceleration/1
  Demux1/2 -> Sum1/2, "Velocity "/2
  Demux/2 -> Sum1/1, "Velocity "/1
  Demux1/1 -> Sum/2, Angle/2
  Demux/1 -> Sum/1, Angle/1
  Sum/1 -> Err1/1
  Sum1/1 -> Err2/1
  Sum2/1 -> Err3/1
  JVA2/1 -> Demux/1, "Encoder "/1
  Ref_JVA2/1 -> Demux1/1, "Ref "/1

== system CtrPlatform_AdaptiveControl/Display/JntVelAccDisplay/Joint3 ==
  JVA3 : Inport
  Ref_JVA3 : Inport  Port=2
  Acceleration : Scope  NumInputPorts=2
      settings: YMin=-5~-5  YMax=5~5  SaveName=ScopeData2
  Angle : Scope  NumInputPorts=2
      settings: TimeRange=10  YMin=-2.999999999999999e-017~-1  YMax=4e-017~1
  Demux : Demux  Outputs=3
  Demux1 : Demux  Outputs=3
  "Encoder " : ToWorkspace  VariableName=EncJVAJ3  SampleTime=-1  SaveFormat=Structure
  Err1 : Scope
      settings: SaveName=ScopeData6
  Err2 : Scope
      settings: SaveName=ScopeData7
  Err3 : Scope
      settings: SaveName=ScopeData8
  "Ref " : ToWorkspace  VariableName=RefJVAJ3  SampleTime=-1  SaveFormat=Structure
  Sum : Sum  Inputs=+|-
  Sum1 : Sum  Inputs=+|-
  Sum2 : Sum  Inputs=+|-
  "Velocity " : Scope  NumInputPorts=2
      settings: YMin=-5~-5  YMax=5~5
  wires:
  Ref_JVA3/1 -> "Ref "/1, Demux1/1
  JVA3/1 -> "Encoder "/1, Demux/1
  Sum2/1 -> Err3/1
  Sum1/1 -> Err2/1
  Sum/1 -> Err1/1
  Demux/1 -> Angle/1, Sum/1
  Demux1/1 -> Angle/2, Sum/2
  Demux/2 -> "Velocity "/1, Sum1/1
  Demux1/2 -> "Velocity "/2, Sum1/2
  Demux/3 -> Acceleration/1, Sum2/1
  Demux1/3 -> Acceleration/2, Sum2/2

== system CtrPlatform_AdaptiveControl/Display/JntVelAccDisplay/Joint4 ==
  JVA4 : Inport
  Ref_JVA4 : Inport  Port=2
  Acceleration : Scope  NumInputPorts=2
      settings: YMin=-5~-5  YMax=5~5  SaveName=ScopeData2
  Angle : Scope  NumInputPorts=2
      settings: TimeRange=10  YMin=-2.999999999999999e-017~-1  YMax=4e-017~1
  Demux : Demux  Outputs=3
  Demux1 : Demux  Outputs=3
  "Encoder " : ToWorkspace  VariableName=EncJVAJ4  SampleTime=-1  SaveFormat=Structure
  Err1 : Scope
      settings: SaveName=ScopeData6
  Err2 : Scope
      settings: SaveName=ScopeData7
  Err3 : Scope
      settings: SaveName=ScopeData8
  "Ref " : ToWorkspace  VariableName=RefJVAJ4  SampleTime=-1  SaveFormat=Structure
  Sum : Sum  Inputs=+|-
  Sum1 : Sum  Inputs=+|-
  Sum2 : Sum  Inputs=+|-
  "Velocity " : Scope  NumInputPorts=2
      settings: YMin=-5~-5  YMax=5~5
  wires:
  Demux1/3 -> Sum2/2, Acceleration/2
  Demux/3 -> Sum2/1, Acceleration/1
  Demux1/2 -> Sum1/2, "Velocity "/2
  Demux/2 -> Sum1/1, "Velocity "/1
  Demux1/1 -> Sum/2, Angle/2
  Demux/1 -> Sum/1, Angle/1
  Sum/1 -> Err1/1
  Sum1/1 -> Err2/1
  Sum2/1 -> Err3/1
  JVA4/1 -> Demux/1, "Encoder "/1
  Ref_JVA4/1 -> Demux1/1, "Ref "/1
